simulink model "EPT"  (R2019b)
settings: Solver=FixedStepDiscrete  StartTime=0.0  StopTime=5  FixedStep=0.005  RelTol=1e-3  EnableMultiTasking=on
PreLoadFcn:
  | try, model_open; catch, disp('Error occurred while executing model pre-load callback: model_open.m'); disp('Please assure that the MATLAB working directory is set to the model directory before opening.'); end
InitFcn:
  | try, model_open; catch, end
undefined symbols (not defined in the file or in its folder): Bridge, GCM, H, ln, raptor_get_param_eval, raptor_get_safe_string, raptor_xcp_function
libraries: Raptor_lib x2810, simulink x374, hdlsllib x19
(part 29 of 45)

== system EPT/Foreground_TimeBase_5ms/CAN/CAN3_exec/20CH_TCS/CH1_CH4_Rx/Convert_Byte2Data2 ==
  HighByte : Inport
  LowByte : Inport  Port=2
  Offset : Inport  Port=3
  Factor : Inport  Port=4
  Add2 : Sum
  Add5 : Sum
  Constant10 : Constant  Value=256
  Data Type Conversion10 : DataTypeConversion  OutDataTypeStr=double
  Divide6 : Product  Inputs=**
  Divide9 : Product  Inputs=**
  Data : Outport  VectorParamsAs1DForOutWhenUnconnected=off
  wires:
  Divide6/1 -> Add2/2
  LowByte/1 -> Add2/1
  Add5/1 -> Data Type Conversion10/1
  HighByte/1 -> Divide6/1
  Constant10/1 -> Divide6/2
  Divide9/1 -> Add5/1
  Add2/1 -> Divide9/1
  Data Type Conversion10/1 -> Data/1
  Factor/1 -> Divide9/2
  Offset/1 -> Add5/2

== system EPT/Foreground_TimeBase_5ms/CAN/CAN3_exec/20CH_TCS/CH1_CH4_Rx/Convert_Byte2Data3 ==
  HighByte : Inport
  LowByte : Inport  Port=2
  Offset : Inport  Port=3
  Factor : Inport  Port=4
  Add2 : Sum
  Add5 : Sum
  Constant10 : Constant  Value=256
  Data Type Conversion10 : DataTypeConversion  OutDataTypeStr=double
  Divide6 : Product  Inputs=**
  Divide9 : Product  Inputs=**
  Data : Outport  VectorParamsAs1DForOutWhenUnconnected=off
  wires:
  Offset/1 -> Add5/2
  Factor/1 -> Divide9/2
  Data Type Conversion10/1 -> Data/1
  Add2/1 -> Divide9/1
  Divide9/1 -> Add5/1
  Constant10/1 -> Divide6/2
  HighByte/1 -> Divide6/1
  Add5/1 -> Data Type Conversion10/1
  LowByte/1 -> Add2/1
  Divide6/1 -> Add2/2

== system EPT/Foreground_TimeBase_5ms/CAN/CAN3_exec/20CH_TCS/CH5_CH8_Rx/Convert_Byte2Data ==
  HighByte : Inport
  LowByte : Inport  Port=2
  Offset : Inport  Port=3
  Factor : Inport  Port=4
  Add2 : Sum
  Add5 : Sum
  Constant10 : Constant  Value=256
  Data Type Conversion10 : DataTypeConversion  OutDataTypeStr=double
  Divide6 : Product  Inputs=**
  Divide9 : Product  Inputs=**
  Data : Outport  VectorParamsAs1DForOutWhenUnconnected=off
  wires:
  Divide6/1 -> Add2/2
  LowByte/1 -> Add2/1
  Add5/1 -> Data Type Conversion10/1
  HighByte/1 -> Divide6/1
  Constant10/1 -> Divide6/2
  Divide9/1 -> Add5/1
  Add2/1 -> Divide9/1
  Data Type Conversion10/1 -> Data/1
  Factor/1 -> Divide9/2
  Offset/1 -> Add5/2

== system EPT/Foreground_TimeBase_5ms/CAN/CAN3_exec/20CH_TCS/CH5_CH8_Rx/Convert_Byte2Data1 ==
  HighByte : Inport
  LowByte : Inport  Port=2
  Offset : Inport  Port=3
  Factor : Inport  Port=4
  Add2 : Sum
  Add5 : Sum
  Constant10 : Constant  Value=256
  Data Type Conversion10 : DataTypeConversion  OutDataTypeStr=double
  Divide6 : Product  Inputs=**
  Divide9 : Product  Inputs=**
  Data : Outport  VectorParamsAs1DForOutWhenUnconnected=off
  wires:
  Offset/1 -> Add5/2
  Factor/1 -> Divide9/2
  Data Type Conversion10/1 -> Data/1
  Add2/1 -> Divide9/1
  Divide9/1 -> Add5/1
  Constant10/1 -> Divide6/2
  HighByte/1 -> Divide6/1
  Add5/1 -> Data Type Conversion10/1
  LowByte/1 -> Add2/1
  Divide6/1 -> Add2/2

== system EPT/Foreground_TimeBase_5ms/CAN/CAN3_exec/20CH_TCS/CH5_CH8_Rx/Convert_Byte2Data2 ==
  HighByte : Inport
  LowByte : Inport  Port=2
  Offset : Inport  Port=3
  Factor : Inport  Port=4
  Add2 : Sum
  Add5 : Sum
  Constant10 : Constant  Value=256
  Data Type Conversion10 : DataTypeConversion  OutDataTypeStr=double
  Divide6 : Product  Inputs=**
  Divide9 : Product  Inputs=**
  Data : Outport  VectorParamsAs1DForOutWhenUnconnected=off
  wires:
  Divide6/1 -> Add2/2
  LowByte/1 -> Add2/1
  Add5/1 -> Data Type Conversion10/1
  HighByte/1 -> Divide6/1
  Constant10/1 -> Divide6/2
  Divide9/1 -> Add5/1
  Add2/1 -> Divide9/1
  Data Type Conversion10/1 -> Data/1
  Factor/1 -> Divide9/2
  Offset/1 -> Add5/2

== system EPT/Foreground_TimeBase_5ms/CAN/CAN3_exec/20CH_TCS/CH5_CH8_Rx/Convert_Byte2Data3 ==
  HighByte : Inport
  LowByte : Inport  Port=2
  Offset : Inport  Port=3
  Factor : Inport  Port=4
  Add2 : Sum
  Add5 : Sum
  Constant10 : Constant  Value=256
  Data Type Conversion10 : DataTypeConversion  OutDataTypeStr=double
  Divide6 : Product  Inputs=**
  Divide9 : Product  Inputs=**
  Data : Outport  VectorParamsAs1DForOutWhenUnconnected=off
  wires:
  Offset/1 -> Add5/2
  Factor/1 -> Divide9/2
  Data Type Conversion10/1 -> Data/1
  Add2/1 -> Divide9/1
  Divide9/1 -> Add5/1
  Constant10/1 -> Divide6/2
  HighByte/1 -> Divide6/1
  Add5/1 -> Data Type Conversion10/1
  LowByte/1 -> Add2/1
  Divide6/1 -> Add2/2

== system EPT/Foreground_TimeBase_5ms/CAN/CAN3_exec/20CH_TCS/CH9_CH12_Rx/Convert_Byte2Data ==
  HighByte : Inport
  LowByte : Inport  Port=2
  Offset : Inport  Port=3
  Factor : Inport  Port=4
  Add2 : Sum
  Add5 : Sum
  Constant10 : Constant  Value=256
  Data Type Conversion10 : DataTypeConversion  OutDataTypeStr=double
  Divide6 : Product  Inputs=**
  Divide9 : Product  Inputs=**
  Data : Outport  VectorParamsAs1DForOutWhenUnconnected=off
  wires:
  Divide6/1 -> Add2/2
  LowByte/1 -> Add2/1
  Add5/1 -> Data Type Conversion10/1
  HighByte/1 -> Divide6/1
  Constant10/1 -> Divide6/2
  Divide9/1 -> Add5/1
  Add2/1 -> Divide9/1
  Data Type Conversion10/1 -> Data/1
  Factor/1 -> Divide9/2
  Offset/1 -> Add5/2

== system EPT/Foreground_TimeBase_5ms/CAN/CAN3_exec/20CH_TCS/CH9_CH12_Rx/Convert_Byte2Data1 ==
  HighByte : Inport
  LowByte : Inport  Port=2
  Offset : Inport  Port=3
  Factor : Inport  Port=4
  Add2 : Sum
  Add5 : Sum
  Constant10 : Constant  Value=256
  Data Type Conversion10 : DataTypeConversion  OutDataTypeStr=double
  Divide6 : Product  Inputs=**
  Divide9 : Product  Inputs=**
  Data : Outport  VectorParamsAs1DForOutWhenUnconnected=off
  wires:
  Offset/1 -> Add5/2
  Factor/1 -> Divide9/2
  Data Type Conversion10/1 -> Data/1
  Add2/1 -> Divide9/1
  Divide9/1 -> Add5/1
  Constant10/1 -> Divide6/2
  HighByte/1 -> Divide6/1
  Add5/1 -> Data Type Conversion10/1
  LowByte/1 -> Add2/1
  Divide6/1 -> Add2/2

== system EPT/Foreground_TimeBase_5ms/CAN/CAN3_exec/20CH_TCS/CH9_CH12_Rx/Convert_Byte2Data2 ==
  HighByte : Inport
  LowByte : Inport  Port=2
  Offset : Inport  Port=3
  Factor : Inport  Port=4
  Add2 : Sum
  Add5 : Sum
  Constant10 : Constant  Value=256
  Data Type Conversion10 : DataTypeConversion  OutDataTypeStr=double
  Divide6 : Product  Inputs=**
  Divide9 : Product  Inputs=**
  Data : Outport  VectorParamsAs1DForOutWhenUnconnected=off
  wires:
  Divide6/1 -> Add2/2
  LowByte/1 -> Add2/1
  Add5/1 -> Data Type Conversion10/1
  HighByte/1 -> Divide6/1
  Constant10/1 -> Divide6/2
  Divide9/1 -> Add5/1
  Add2/1 -> Divide9/1
  Data Type Conversion10/1 -> Data/1
  Factor/1 -> Divide9/2
  Offset/1 -> Add5/2

== system EPT/Foreground_TimeBase_5ms/CAN/CAN3_exec/20CH_TCS/CH9_CH12_Rx/Convert_Byte2Data3 ==
  HighByte : Inport
  LowByte : Inport  Port=2
  Offset : Inport  Port=3
  Factor : Inport  Port=4
  Add2 : Sum
  Add5 : Sum
  Constant10 : Constant  Value=256
  Data Type Conversion10 : DataTypeConversion  OutDataTypeStr=double
  Divide6 : Product  Inputs=**
  Divide9 : Product  Inputs=**
  Data : Outport  VectorParamsAs1DForOutWhenUnconnected=off
  wires:
  Offset/1 -> Add5/2
  Factor/1 -> Divide9/2
  Data Type Conversion10/1 -> Data/1
  Add2/1 -> Divide9/1
  Divide9/1 -> Add5/1
  Constant10/1 -> Divide6/2
  HighByte/1 -> Divide6/1
  Add5/1 -> Data Type Conversion10/1
  LowByte/1 -> Add2/1
  Divide6/1 -> Add2/2

== system EPT/Foreground_TimeBase_5ms/CAN/CAN3_exec/20CH_TCS/CountTrigger/CycleTrigger ==
  In1 : Inport
  In2 : Inport  Port=2
  Add : Sum
  Add1 : Sum
  Add2 : Sum  Inputs=+-
  Constant1 : Constant
  Constant2 : Constant  Value=0
  Constant3 : Constant
  Data Type Conversion1 : DataTypeConversion
  Data Type Conversion2 : DataTypeConversion
  Display : Display
  Relational Operator1 : RelationalOperator  OutDataTypeStr=boolean  RndMeth=Simplest
  Scope : Scope
  Scope1 : Scope
  Scope2 : Scope
  Switch : Switch  Threshold=1
  Unit Delay : UnitDelay  SampleTime=-1  HasFrameUpgradeWarning=on
  Unit Delay1 : UnitDelay  SampleTime=-1  HasFrameUpgradeWarning=on
  Trigger : Outport  VectorParamsAs1DForOutWhenUnconnected=off
  wires:
  Constant3/1 -> Add2/2
  In2/1 -> Add2/1
  Add2/1 -> Data Type Conversion1/1
  Data Type Conversion2/1 -> Switch/2, Add/2
  Constant2/1 -> Switch/3
  Data Type Conversion1/1 -> Relational Operator1/2
  Relational Operator1/1 -> Trigger/1, Scope2/1
  Constant1/1 -> Add1/2
  Unit Delay1/1 -> Add1/1
  Add1/1 -> Display/1, Unit Delay1/1, Scope/1
  Switch/1 -> Unit Delay/1, Scope1/1, Relational Operator1/1
  Unit Delay/1 -> Add/1
  In1/1 -> Data Type Conversion2/1
  Add/1 -> Switch/1

== system EPT/Foreground_TimeBase_5ms/CAN/CAN3_exec/DCDC/CountTrigger/CycleTrigger ==
  In1 : Inport
  In2 : Inport  Port=2
  Add : Sum
  Add1 : Sum
  Add2 : Sum  Inputs=+-
  Constant1 : Constant
  Constant2 : Constant  Value=0
  Constant3 : Constant
  Data Type Conversion1 : DataTypeConversion
  Data Type Conversion2 : DataTypeConversion
  Display : Display
  Relational Operator1 : RelationalOperator  OutDataTypeStr=boolean  RndMeth=Simplest
  Scope : Scope
  Scope1 : Scope
  Scope2 : Scope
  Switch : Switch  Threshold=1
  Unit Delay : UnitDelay  SampleTime=-1  HasFrameUpgradeWarning=on
  Unit Delay1 : UnitDelay  SampleTime=-1  HasFrameUpgradeWarning=on
  Trigger : Outport  VectorParamsAs1DForOutWhenUnconnected=off
  wires:
  Constant3/1 -> Add2/2
  In2/1 -> Add2/1
  Add2/1 -> Data Type Conversion1/1
  Data Type Conversion2/1 -> Switch/2, Add/2
  Constant2/1 -> Switch/3
  Data Type Conversion1/1 -> Relational Operator1/2
  Relational Operator1/1 -> Trigger/1, Scope2/1
  Constant1/1 -> Add1/2
  Unit Delay1/1 -> Add1/1
  Add1/1 -> Display/1, Unit Delay1/1, Scope/1
  Switch/1 -> Unit Delay/1, Scope1/1, Relational Operator1/1
  Unit Delay/1 -> Add/1
  In1/1 -> Data Type Conversion2/1
  Add/1 -> Switch/1

== system EPT/Foreground_TimeBase_5ms/CAN/CAN3_exec/DCDC/DCDC_RX_0x180XF45D /Convert_Byte2Data1 ==
  HighByte : Inport
  LowByte : Inport  Port=2
  Offset : Inport  Port=3
  Factor : Inport  Port=4
  Add2 : Sum
  Add5 : Sum
  Constant10 : Constant  Value=256
  Data Type Conversion10 : DataTypeConversion  OutDataTypeStr=double
  Divide6 : Product  Inputs=**
  Divide9 : Product  Inputs=**
  Data : Outport  VectorParamsAs1DForOutWhenUnconnected=off
  wires:
  Offset/1 -> Add5/2
  Factor/1 -> Divide9/2
  Data Type Conversion10/1 -> Data/1
  Add2/1 -> Divide9/1
  Divide9/1 -> Add5/1
  Constant10/1 -> Divide6/2
  HighByte/1 -> Divide6/1
  Add5/1 -> Data Type Conversion10/1
  LowByte/1 -> Add2/1
  Divide6/1 -> Add2/2

== system EPT/Foreground_TimeBase_5ms/CAN/CAN3_exec/DCDC/DCDC_RX_0x180XF45D /Convert_Byte2Data2 ==
  HighByte : Inport
  LowByte : Inport  Port=2
  Offset : Inport  Port=3
  Factor : Inport  Port=4
  Add2 : Sum
  Add5 : Sum
  Constant10 : Constant  Value=256
  Data Type Conversion10 : DataTypeConversion  OutDataTypeStr=double
  Divide6 : Product  Inputs=**
  Divide9 : Product  Inputs=**
  Data : Outport  VectorParamsAs1DForOutWhenUnconnected=off
  wires:
  Divide6/1 -> Add2/2
  LowByte/1 -> Add2/1
  Add5/1 -> Data Type Conversion10/1
  HighByte/1 -> Divide6/1
  Constant10/1 -> Divide6/2
  Divide9/1 -> Add5/1
  Add2/1 -> Divide9/1
  Data Type Conversion10/1 -> Data/1
  Factor/1 -> Divide9/2
  Offset/1 -> Add5/2

== system EPT/Foreground_TimeBase_5ms/CAN/CAN3_exec/DCDC/DCDC_RX_0x180XF45D /Convert_Byte2Data3 ==
  HighByte : Inport
  LowByte : Inport  Port=2
  Offset : Inport  Port=3
  Factor : Inport  Port=4
  Add2 : Sum
  Add5 : Sum
  Constant10 : Constant  Value=256
  Data Type Conversion10 : DataTypeConversion  OutDataTypeStr=double
  Divide6 : Product  Inputs=**
  Divide9 : Product  Inputs=**
  Data : Outport  VectorParamsAs1DForOutWhenUnconnected=off
  wires:
  Divide6/1 -> Add2/2
  LowByte/1 -> Add2/1
  Add5/1 -> Data Type Conversion10/1
  HighByte/1 -> Divide6/1
  Constant10/1 -> Divide6/2
  Divide9/1 -> Add5/1
  Add2/1 -> Divide9/1
  Data Type Conversion10/1 -> Data/1
  Factor/1 -> Divide9/2
  Offset/1 -> Add5/2

== system EPT/Foreground_TimeBase_5ms/CAN/CAN3_exec/HyPer9_MCU/CountTrigger2/CycleTrigger ==
  In1 : Inport
  In2 : Inport  Port=2
  Add : Sum
  Add1 : Sum
  Add2 : Sum  Inputs=+-
  Constant1 : Constant
  Constant2 : Constant  Value=0
  Constant3 : Constant
  Data Type Conversion1 : DataTypeConversion
  Data Type Conversion2 : DataTypeConversion
  Display : Display
  Relational Operator1 : RelationalOperator  OutDataTypeStr=boolean  RndMeth=Simplest
  Scope : Scope
  Scope1 : Scope
  Scope2 : Scope
  Switch : Switch  Threshold=1
  Unit Delay : UnitDelay  SampleTime=-1  HasFrameUpgradeWarning=on
  Unit Delay1 : UnitDelay  SampleTime=-1  HasFrameUpgradeWarning=on
  Trigger : Outport  VectorParamsAs1DForOutWhenUnconnected=off
  wires:
  Add/1 -> Switch/1
  In1/1 -> Data Type Conversion2/1
  Unit Delay/1 -> Add/1
  Switch/1 -> Relational Operator1/1, Scope1/1, Unit Delay/1
  Add1/1 -> Scope/1, Unit Delay1/1, Display/1
  Unit Delay1/1 -> Add1/1
  Constant1/1 -> Add1/2
  Relational Operator1/1 -> Scope2/1, Trigger/1
  Data Type Conversion1/1 -> Relational Operator1/2
  Constant2/1 -> Switch/3
  Data Type Conversion2/1 -> Add/2, Switch/2
  Add2/1 -> Data Type Conversion1/1
  In2/1 -> Add2/1
  Constant3/1 -> Add2/2

== system EPT/Foreground_TimeBase_5ms/CAN/CAN3_exec/HyPer9_MCU/RPDO1/Byte1 ==
  Bit Shift1 : hdlsllib/Logic and Bit Operations/Bit Shift  mode=Shift Left Logical  N=1
  Bit Shift2 : hdlsllib/Logic and Bit Operations/Bit Shift  mode=Shift Left Logical  N=2
  Bit Shift3 : hdlsllib/Logic and Bit Operations/Bit Shift  mode=Shift Left Logical  N=3
  Bit Shift4 : hdlsllib/Logic and Bit Operations/Bit Shift  mode=Shift Left Logical  N=4
  Bit Shift5 : hdlsllib/Logic and Bit Operations/Bit Shift  mode=Shift Left Logical  N=5
  Bit Shift6 : hdlsllib/Logic and Bit Operations/Bit Shift  mode=Shift Left Logical  N=6
  Bit Shift7 : hdlsllib/Logic and Bit Operations/Bit Shift  mode=Shift Left Logical  N=7
  Bitwise OR : simulink/Logic and Bit Operations/Bitwise Operator  logicop=OR  UseBitMask=off  NumInputPorts=8  BitMask=bin2dec('11011001')  BitMaskRealWorld=Stored Integer
  Data Type Conversion{1..9} (9 alike) : DataTypeConversion  OutDataTypeStr=uint8
  "First Sw Reset Request " : Constant  Value=0  OutDataTypeStr=uint8
  IsPositive{1..7} (7 alike) : simulink/Logic and Bit Operations/Compare To Zero  relop=>  OutDataTypeStr=boolean
  Request for Digital Output 1 : Constant  Value=0  OutDataTypeStr=uint8
  Request for Digital Output 2 : Constant  Value=0  OutDataTypeStr=uint8
  Request for Driver Output 1 in Voltage Mode : Constant  Value=0  OutDataTypeStr=uint8
  Request for Driver Output 2 in Voltage Mode : Constant  Value=0  OutDataTypeStr=uint8
  Request for Driver Output 3 in Voltage Mode : Constant  Value=0  OutDataTypeStr=uint8
  Request for Driver Output 4 in Voltage Mode (only Control Mode allowed) : Constant  Value=0  OutDataTypeStr=uint8
  Second Sw Reset Request : Constant  Value=0  OutDataTypeStr=uint8
  Byte : Outport
  wires:
  IsPositive6/1 -> Data Type Conversion7/1
  Request for Driver Output 4 in Voltage Mode (only Control Mode allowed)/1 -> IsPositive7/1
  Data Type Conversion2/1 -> Bitwise OR/1
  IsPositive7/1 -> Data Type Conversion8/1
  IsPositive3/1 -> Data Type Conversion4/1
  Request for Driver Output 1 in Voltage Mode/1 -> IsPositive2/1
  Bit Shift4/1 -> Bitwise OR/5
  Bit Shift6/1 -> Bitwise OR/7
  IsPositive2/1 -> Data Type Conversion3/1
  "First Sw Reset Request "/1 -> IsPositive5/1
  IsPositive5/1 -> Data Type Conversion6/1
  Bit Shift3/1 -> Bitwise OR/4
  Data Type Conversion5/1 -> Bit Shift4/1
  Data Type Conversion8/1 -> Bit Shift7/1
  Bit Shift7/1 -> Bitwise OR/8
  Request for Digital Output 1/1 -> Data Type Conversion2/1
  Bit Shift2/1 -> Bitwise OR/3
  Bitwise OR/1 -> Data Type Conversion9/1
  Data Type Conversion4/1 -> Bit Shift3/1
  Request for Digital Output 2/1 -> IsPositive1/1
  Data Type Conversion7/1 -> Bit Shift6/1
  IsPositive1/1 -> Data Type Conversion1/1
  Data Type Conversion1/1 -> Bit Shift1/1
  Bit Shift5/1 -> Bitwise OR/6
  Request for Driver Output 2 in Voltage Mode/1 -> IsPositive3/1
  Second Sw Reset Request/1 -> IsPositive6/1
  IsPositive4/1 -> Data Type Conversion5/1
  Request for Driver Output 3 in Voltage Mode/1 -> IsPositive4/1
  Data Type Conversion9/1 -> Byte/1
  Data Type Conversion6/1 -> Bit Shift5/1
  Bit Shift1/1 -> Bitwise OR/2
  Data Type Conversion3/1 -> Bit Shift2/1

== system EPT/Foreground_TimeBase_5ms/CAN/CAN3_exec/HyPer9_MCU/RPDO1/Convert_Data2Byte ==
  Data : Inport
  Factor : Inport  Port=2
  Offset : Inport  Port=3
  Add : Sum
  Bitwise Operator : simulink/Logic and Bit Operations/Bitwise Operator  logicop=AND  UseBitMask=on  BitMask=bin2dec('1111111100000000')  BitMaskRealWorld=Stored Integer
  Bitwise Operator1 : simulink/Logic and Bit Operations/Bitwise Operator  logicop=AND  UseBitMask=on  BitMask=bin2dec('0000000011111111')  BitMaskRealWorld=Stored Integer
  Compare To Zero : simulink/Logic and Bit Operations/Compare To Zero  relop=~=  OutDataTypeStr=boolean
  Constant : Constant
  Data Type Conversion : DataTypeConversion
  Data Type Conversion1 : DataTypeConversion  OutDataTypeStr=uint16
  Data Type Conversion2 : DataTypeConversion
  Display : Display
      settings: Format=hex (Stored Integer)
  Divide : Product  Inputs=**
  Shift Arithmetic : ArithShift  BitShiftNumber=8  BitShiftDirection=Right
  Switch : Switch  Criteria=u2 > Threshold
  LowByte : Outport  VectorParamsAs1DForOutWhenUnconnected=off
  HighByte : Outport  Port=2  VectorParamsAs1DForOutWhenUnconnected=off
  wires:
  Compare To Zero/1 -> Switch/2
  Factor/1 -> Switch/1, Compare To Zero/1
  Data Type Conversion2/1 -> HighByte/1
  Data Type Conversion/1 -> LowByte/1
  Constant/1 -> Switch/3
  Switch/1 -> Divide/2
  Bitwise Operator/1 -> Shift Arithmetic/1
  Offset/1 -> Add/2
  Shift Arithmetic/1 -> Data Type Conversion2/1
  Bitwise Operator1/1 -> Data Type Conversion/1
  Data Type Conversion1/1 -> Bitwise Operator/1, Display/1, Bitwise Operator1/1
  Divide/1 -> Add/1
  Data/1 -> Divide/1
  Add/1 -> Data Type Conversion1/1

== system EPT/Foreground_TimeBase_5ms/CAN/CAN3_exec/HyPer9_MCU/RPDO1/Convert_Data2Byte1 ==
  Data : Inport
  Factor : Inport  Port=2
  Offset : Inport  Port=3
  Add : Sum
  Bitwise Operator : simulink/Logic and Bit Operations/Bitwise Operator  logicop=AND  UseBitMask=on  BitMask=bin2dec('1111111100000000')  BitMaskRealWorld=Stored Integer
  Bitwise Operator1 : simulink/Logic and Bit Operations/Bitwise Operator  logicop=AND  UseBitMask=on  BitMask=bin2dec('0000000011111111')  BitMaskRealWorld=Stored Integer
  Compare To Zero : simulink/Logic and Bit Operations/Compare To Zero  relop=~=  OutDataTypeStr=boolean
  Constant : Constant
  Data Type Conversion : DataTypeConversion
  Data Type Conversion1 : DataTypeConversion  OutDataTypeStr=uint16
  Data Type Conversion2 : DataTypeConversion
  Display : Display
      settings: Format=hex (Stored Integer)
  Divide : Product  Inputs=**
  Shift Arithmetic : ArithShift  BitShiftNumber=8  BitShiftDirection=Right
  Switch : Switch  Criteria=u2 > Threshold
  LowByte : Outport  VectorParamsAs1DForOutWhenUnconnected=off
  HighByte : Outport  Port=2  VectorParamsAs1DForOutWhenUnconnected=off
  wires:
  Add/1 -> Data Type Conversion1/1
  Data/1 -> Divide/1
  Divide/1 -> Add/1
  Data Type Conversion1/1 -> Bitwise Operator1/1, Display/1, Bitwise Operator/1
  Bitwise Operator1/1 -> Data Type Conversion/1
  Shift Arithmetic/1 -> Data Type Conversion2/1
  Offset/1 -> Add/2
  Bitwise Operator/1 -> Shift Arithmetic/1
  Switch/1 -> Divide/2
  Constant/1 -> Switch/3
  Data Type Conversion/1 -> LowByte/1
  Data Type Conversion2/1 -> HighByte/1
  Factor/1 -> Compare To Zero/1, Switch/1
  Compare To Zero/1 -> Switch/2

== system EPT/Foreground_TimeBase_5ms/CAN/CAN3_exec/HyPer9_MCU/RPDO1/Convert_Data2Byte2 ==
  Data : Inport
  Factor : Inport  Port=2
  Offset : Inport  Port=3
  Add : Sum
  Bitwise Operator : simulink/Logic and Bit Operations/Bitwise Operator  logicop=AND  UseBitMask=on  BitMask=bin2dec('1111111100000000')  BitMaskRealWorld=Stored Integer
  Bitwise Operator1 : simulink/Logic and Bit Operations/Bitwise Operator  logicop=AND  UseBitMask=on  BitMask=bin2dec('0000000011111111')  BitMaskRealWorld=Stored Integer
  Compare To Zero : simulink/Logic and Bit Operations/Compare To Zero  relop=~=  OutDataTypeStr=boolean
  Constant : Constant
  Data Type Conversion : DataTypeConversion
  Data Type Conversion1 : DataTypeConversion  OutDataTypeStr=uint16
  Data Type Conversion2 : DataTypeConversion
  Display : Display
      settings: Format=hex (Stored Integer)
  Divide : Product  Inputs=**
  Shift Arithmetic : ArithShift  BitShiftNumber=8  BitShiftDirection=Right
  Switch : Switch  Criteria=u2 > Threshold
  LowByte : Outport  VectorParamsAs1DForOutWhenUnconnected=off
  HighByte : Outport  Port=2  VectorParamsAs1DForOutWhenUnconnected=off
  wires:
  Compare To Zero/1 -> Switch/2
  Factor/1 -> Switch/1, Compare To Zero/1
  Data Type Conversion2/1 -> HighByte/1
  Data Type Conversion/1 -> LowByte/1
  Constant/1 -> Switch/3
  Switch/1 -> Divide/2
  Bitwise Operator/1 -> Shift Arithmetic/1
  Offset/1 -> Add/2
  Shift Arithmetic/1 -> Data Type Conversion2/1
  Bitwise Operator1/1 -> Data Type Conversion/1
  Data Type Conversion1/1 -> Bitwise Operator/1, Display/1, Bitwise Operator1/1
  Divide/1 -> Add/1
  Data/1 -> Divide/1
  Add/1 -> Data Type Conversion1/1

== system EPT/Foreground_TimeBase_5ms/CAN/CAN3_exec/HyPer9_MCU/RPDO2/Byte5 ==
  Bit Shift1 : hdlsllib/Logic and Bit Operations/Bit Shift  mode=Shift Left Logical  N=2
  Bit Shift2 : hdlsllib/Logic and Bit Operations/Bit Shift  mode=Shift Left Logical  N=3
  Bit Shift3 : hdlsllib/Logic and Bit Operations/Bit Shift  mode=Shift Left Logical  N=4
  Bit Shift4 : hdlsllib/Logic and Bit Operations/Bit Shift  mode=Shift Left Logical  N=5
  Bit Shift5 : hdlsllib/Logic and Bit Operations/Bit Shift  mode=Shift Left Logical  N=6
  Bitwise Operator1 : simulink/Logic and Bit Operations/Bitwise Operator  logicop=AND  UseBitMask=on  BitMask=bin2dec('11')  BitMaskRealWorld=Stored Integer
  Bitwise OR : simulink/Logic and Bit Operations/Bitwise Operator  logicop=OR  UseBitMask=off  NumInputPorts=6  BitMask=bin2dec('11011001')  BitMaskRealWorld=Stored Integer
  Data Type Conversion{1..6,9} (7 alike) : DataTypeConversion  OutDataTypeStr=uint8
  Display : Display
      settings: Format=binary (Stored Integer)
  IsPositive{1..5} (5 alike) : simulink/Logic and Bit Operations/Compare To Zero  relop=>  OutDataTypeStr=boolean
  "Motor 1 - Control Mode Request " : Constant  Value=2  OutDataTypeStr=uint8
  raptor_adjustment : Raptor_lib/Data Storage/raptor_adjustment  paramName='Cal_Motor1_Motor1_PWM_Output_Enable_Request'  nameSource=Parameter  initValue=0.00  dataType=double  storage=Calibration  calDispType=Number  calEnum={'False', 'True'}  calGain=1.0  calOffset=0.0  calMax=9  calMin=-inf  calFormat='-1'  calUnit=''  calHelp=''  calAccess=1  calFunction=raptor_xcp_function(gcb)  calDispHeaders=off  calColHeaders={'Col1' 'Col2' 'Col3'}  calRowHeaders={'Row1' 'Row2' 'Row3'}
      settings: SourceProductName=Raptor
  raptor_adjustment1 : Raptor_lib/Data Storage/raptor_adjustment  paramName='Cal_Motor1_Reference_Torque_Enable_Request'  nameSource=Parameter  initValue=0.00  dataType=double  storage=Calibration  calDispType=Number  calEnum={'False', 'True'}  calGain=1.0  calOffset=0.0  calMax=9  calMin=-inf  calFormat='-1'  calUnit=''  calHelp=''  calAccess=1  calFunction=raptor_xcp_function(gcb)  calDispHeaders=off  calColHeaders={'Col1' 'Col2' 'Col3'}  calRowHeaders={'Row1' 'Row2' 'Row3'}
      settings: SourceProductName=Raptor
  raptor_adjustment2 : Raptor_lib/Data Storage/raptor_adjustment  paramName='Cal_Motor1_Emergency_Stop_Request'  nameSource=Parameter  initValue=0.00  dataType=double  storage=Calibration  calDispType=Number  calEnum={'False', 'True'}  calGain=1.0  calOffset=0.0  calMax=9  calMin=-inf  calFormat='-1'  calUnit=''  calHelp=''  calAccess=1  calFunction=raptor_xcp_function(gcb)  calDispHeaders=off  calColHeaders={'Col1' 'Col2' 'Col3'}  calRowHeaders={'Row1' 'Row2' 'Row3'}
      settings: SourceProductName=Raptor
  raptor_adjustment3 : Raptor_lib/Data Storage/raptor_adjustment  paramName='Cal_Motor1_Safe_Stop_Request'  nameSource=Parameter  initValue=0.00  dataType=double  storage=Calibration  calDispType=Number  calEnum={'False', 'True'}  calGain=1.0  calOffset=0.0  calMax=9  calMin=-inf  calFormat='-1'  calUnit=''  calHelp=''  calAccess=1  calFunction=raptor_xcp_function(gcb)  calDispHeaders=off  calColHeaders={'Col1' 'Col2' 'Col3'}  calRowHeaders={'Row1' 'Row2' 'Row3'}
      settings: SourceProductName=Raptor
  raptor_adjustment4 : Raptor_lib/Data Storage/raptor_adjustment  paramName='Cal_Motor1_Speed_Limit_Request'  nameSource=Parameter  initValue=0.00  dataType=double  storage=Calibration  calDispType=Number  calEnum={'False', 'True'}  calGain=1.0  calOffset=0.0  calMax=9  calMin=-inf  calFormat='-1'  calUnit=''  calHelp=''  calAccess=1  calFunction=raptor_xcp_function(gcb)  calDispHeaders=off  calColHeaders={'Col1' 'Col2' 'Col3'}  calRowHeaders={'Row1' 'Row2' 'Row3'}
      settings: SourceProductName=Raptor
  Byte : Outport
  wires:
  Data Type Conversion2/1 -> Bitwise OR/1
  IsPositive3/1 -> Data Type Conversion4/1
  raptor_adjustment1/1 -> IsPositive2/1
  Bit Shift4/1 -> Bitwise OR/5
  IsPositive2/1 -> Data Type Conversion3/1
  raptor_adjustment4/1 -> IsPositive5/1
  IsPositive5/1 -> Data Type Conversion6/1
  Bit Shift3/1 -> Bitwise OR/4
  Data Type Conversion5/1 -> Bit Shift4/1
  "Motor 1 - Control Mode Request "/1 -> Bitwise Operator1/1
  Bit Shift2/1 -> Bitwise OR/3
  Bitwise OR/1 -> Data Type Conversion9/1
  Data Type Conversion4/1 -> Bit Shift3/1
  raptor_adjustment/1 -> IsPositive1/1
  IsPositive1/1 -> Data Type Conversion1/1
  Data Type Conversion1/1 -> Bit Shift1/1
  Bit Shift5/1 -> Bitwise OR/6
  raptor_adjustment2/1 -> IsPositive3/1
  IsPositive4/1 -> Data Type Conversion5/1
  raptor_adjustment3/1 -> IsPositive4/1
  Data Type Conversion9/1 -> Display/1, Byte/1
  Data Type Conversion6/1 -> Bit Shift5/1
  Bit Shift1/1 -> Bitwise OR/2
  Data Type Conversion3/1 -> Bit Shift2/1
  Bitwise Operator1/1 -> Data Type Conversion2/1

== system EPT/Foreground_TimeBase_5ms/CAN/CAN3_exec/HyPer9_MCU/RPDO2/Convert_Data2Byte ==
  Data : Inport
  Factor : Inport  Port=2
  Offset : Inport  Port=3
  Add : Sum
  Bitwise Operator : simulink/Logic and Bit Operations/Bitwise Operator  logicop=AND  UseBitMask=on  BitMask=bin2dec('1111111100000000')  BitMaskRealWorld=Stored Integer
  Bitwise Operator1 : simulink/Logic and Bit Operations/Bitwise Operator  logicop=AND  UseBitMask=on  BitMask=bin2dec('0000000011111111')  BitMaskRealWorld=Stored Integer
  Compare To Zero : simulink/Logic and Bit Operations/Compare To Zero  relop=~=  OutDataTypeStr=boolean
  Constant : Constant
  Data Type Conversion : DataTypeConversion
  Data Type Conversion1 : DataTypeConversion  OutDataTypeStr=uint16
  Data Type Conversion2 : DataTypeConversion
  Display : Display
      settings: Format=hex (Stored Integer)
  Divide : Product  Inputs=**
  Shift Arithmetic : ArithShift  BitShiftNumber=8  BitShiftDirection=Right
  Switch : Switch  Criteria=u2 > Threshold
  LowByte : Outport  VectorParamsAs1DForOutWhenUnconnected=off
  HighByte : Outport  Port=2  VectorParamsAs1DForOutWhenUnconnected=off
  wires:
  Add/1 -> Data Type Conversion1/1
  Data/1 -> Divide/1
  Divide/1 -> Add/1
  Data Type Conversion1/1 -> Bitwise Operator1/1, Display/1, Bitwise Operator/1
  Bitwise Operator1/1 -> Data Type Conversion/1
  Shift Arithmetic/1 -> Data Type Conversion2/1
  Offset/1 -> Add/2
  Bitwise Operator/1 -> Shift Arithmetic/1
  Switch/1 -> Divide/2
  Constant/1 -> Switch/3
  Data Type Conversion/1 -> LowByte/1
  Data Type Conversion2/1 -> HighByte/1
  Factor/1 -> Compare To Zero/1, Switch/1
  Compare To Zero/1 -> Switch/2

== system EPT/Foreground_TimeBase_5ms/CAN/CAN3_exec/HyPer9_MCU/RPDO2/Convert_Data2Byte1 ==
  Data : Inport
  Factor : Inport  Port=2
  Offset : Inport  Port=3
  Add : Sum
  Bitwise Operator : simulink/Logic and Bit Operations/Bitwise Operator  logicop=AND  UseBitMask=on  BitMask=bin2dec('1111111100000000')  BitMaskRealWorld=Stored Integer
  Bitwise Operator1 : simulink/Logic and Bit Operations/Bitwise Operator  logicop=AND  UseBitMask=on  BitMask=bin2dec('0000000011111111')  BitMaskRealWorld=Stored Integer
  Compare To Zero : simulink/Logic and Bit Operations/Compare To Zero  relop=~=  OutDataTypeStr=boolean
  Constant : Constant
  Data Type Conversion : DataTypeConversion
  Data Type Conversion1 : DataTypeConversion  OutDataTypeStr=uint16
  Data Type Conversion2 : DataTypeConversion
  Display : Display
      settings: Format=hex (Stored Integer)
  Divide : Product  Inputs=**
  Shift Arithmetic : ArithShift  BitShiftNumber=8  BitShiftDirection=Right
  Switch : Switch  Criteria=u2 > Threshold
  LowByte : Outport  VectorParamsAs1DForOutWhenUnconnected=off
  HighByte : Outport  Port=2  VectorParamsAs1DForOutWhenUnconnected=off
  wires:
  Compare To Zero/1 -> Switch/2
  Factor/1 -> Switch/1, Compare To Zero/1
  Data Type Conversion2/1 -> HighByte/1
  Data Type Conversion/1 -> LowByte/1
  Constant/1 -> Switch/3
  Switch/1 -> Divide/2
  Bitwise Operator/1 -> Shift Arithmetic/1
  Offset/1 -> Add/2
  Shift Arithmetic/1 -> Data Type Conversion2/1
  Bitwise Operator1/1 -> Data Type Conversion/1
  Data Type Conversion1/1 -> Bitwise Operator/1, Display/1, Bitwise Operator1/1
  Divide/1 -> Add/1
  Data/1 -> Divide/1
  Add/1 -> Data Type Conversion1/1

== system EPT/Foreground_TimeBase_5ms/CAN/CAN3_exec/HyPer9_MCU/RPDO2/Convert_Data2Byte2 ==
  Data : Inport
  Factor : Inport  Port=2
  Offset : Inport  Port=3
  Add : Sum
  Bitwise Operator1 : simulink/Logic and Bit Operations/Bitwise Operator  logicop=AND  UseBitMask=on  BitMask=bin2dec('0000000011111111')  BitMaskRealWorld=Stored Integer
  Compare To Zero : simulink/Logic and Bit Operations/Compare To Zero  relop=~=  OutDataTypeStr=boolean
  Constant : Constant
  Data Type Conversion : DataTypeConversion
  Data Type Conversion1 : DataTypeConversion  OutDataTypeStr=uint16
  Display : Display
      settings: Format=hex (Stored Integer)
  Divide : Product  Inputs=**
  Switch : Switch  Criteria=u2 > Threshold
  LowByte : Outport  VectorParamsAs1DForOutWhenUnconnected=off
  wires:
  Add/1 -> Data Type Conversion1/1
  Data/1 -> Divide/1
  Divide/1 -> Add/1
  Data Type Conversion1/1 -> Display/1, Bitwise Operator1/1
  Bitwise Operator1/1 -> Data Type Conversion/1
  Offset/1 -> Add/2
  Switch/1 -> Divide/2
  Constant/1 -> Switch/3
  Data Type Conversion/1 -> LowByte/1
  Factor/1 -> Compare To Zero/1, Switch/1
  Compare To Zero/1 -> Switch/2

== system EPT/Foreground_TimeBase_5ms/CAN/CAN3_exec/HyPer9_MCU/RPDO3/Byte5 ==
  Bit Shift1 : hdlsllib/Logic and Bit Operations/Bit Shift  mode=Shift Left Logical  N=2
  Bit Shift2 : hdlsllib/Logic and Bit Operations/Bit Shift  mode=Shift Left Logical  N=3
  Bit Shift3 : hdlsllib/Logic and Bit Operations/Bit Shift  mode=Shift Left Logical  N=4
  Bit Shift4 : hdlsllib/Logic and Bit Operations/Bit Shift  mode=Shift Left Logical  N=5
  Bit Shift5 : hdlsllib/Logic and Bit Operations/Bit Shift  mode=Shift Left Logical  N=6
  Bitwise Operator1 : simulink/Logic and Bit Operations/Bitwise Operator  logicop=AND  UseBitMask=on  BitMask=bin2dec('11')  BitMaskRealWorld=Stored Integer
  Bitwise OR : simulink/Logic and Bit Operations/Bitwise Operator  logicop=OR  UseBitMask=off  NumInputPorts=6  BitMask=bin2dec('11011001')  BitMaskRealWorld=Stored Integer
  Data Type Conversion{1..6,9} (7 alike) : DataTypeConversion  OutDataTypeStr=uint8
  Display : Display
      settings: Format=binary (Stored Integer)
  IsPositive{1..5} (5 alike) : simulink/Logic and Bit Operations/Compare To Zero  relop=>  OutDataTypeStr=boolean
  "Motor 2 - Control Mode Request " : Constant  Value=0  OutDataTypeStr=uint8
  "Motor 2 - Emergency Stop Request " : Constant  Value=0  OutDataTypeStr=uint8
  "Motor 2 - PWM Output Enable Request " : Constant  Value=0  OutDataTypeStr=uint8
  "Motor 2 - Reference Speed/Torque Enable Request " : Constant  Value=0  OutDataTypeStr=uint8
  "Motor 2 - Safe Stop Request " : Constant  Value=0  OutDataTypeStr=uint8
  "Motor 2 - Speed Limit Request " : Constant  Value=0  OutDataTypeStr=uint8
  Byte : Outport
  wires:
  Bitwise Operator1/1 -> Data Type Conversion2/1
  Data Type Conversion3/1 -> Bit Shift2/1
  Bit Shift1/1 -> Bitwise OR/2
  Data Type Conversion6/1 -> Bit Shift5/1
  Data Type Conversion9/1 -> Byte/1, Display/1
  "Motor 2 - Safe Stop Request "/1 -> IsPositive4/1
  IsPositive4/1 -> Data Type Conversion5/1
  "Motor 2 - Emergency Stop Request "/1 -> IsPositive3/1
  Bit Shift5/1 -> Bitwise OR/6
  Data Type Conversion1/1 -> Bit Shift1/1
  IsPositive1/1 -> Data Type Conversion1/1
  "Motor 2 - PWM Output Enable Request "/1 -> IsPositive1/1
  Data Type Conversion4/1 -> Bit Shift3/1
  Bitwise OR/1 -> Data Type Conversion9/1
  Bit Shift2/1 -> Bitwise OR/3
  "Motor 2 - Control Mode Request "/1 -> Bitwise Operator1/1
  Data Type Conversion5/1 -> Bit Shift4/1
  Bit Shift3/1 -> Bitwise OR/4
  IsPositive5/1 -> Data Type Conversion6/1
  "Motor 2 - Speed Limit Request "/1 -> IsPositive5/1
  IsPositive2/1 -> Data Type Conversion3/1
  Bit Shift4/1 -> Bitwise OR/5
  "Motor 2 - Reference Speed/Torque Enable Request "/1 -> IsPositive2/1
  IsPositive3/1 -> Data Type Conversion4/1
  Data Type Conversion2/1 -> Bitwise OR/1

== system EPT/Foreground_TimeBase_5ms/CAN/CAN3_exec/HyPer9_MCU/RPDO3/Convert_Data2Byte ==
  Data : Inport
  Factor : Inport  Port=2
  Offset : Inport  Port=3
  Add : Sum
  Bitwise Operator : simulink/Logic and Bit Operations/Bitwise Operator  logicop=AND  UseBitMask=on  BitMask=bin2dec('1111111100000000')  BitMaskRealWorld=Stored Integer
  Bitwise Operator1 : simulink/Logic and Bit Operations/Bitwise Operator  logicop=AND  UseBitMask=on  BitMask=bin2dec('0000000011111111')  BitMaskRealWorld=Stored Integer
  Compare To Zero : simulink/Logic and Bit Operations/Compare To Zero  relop=~=  OutDataTypeStr=boolean
  Constant : Constant
  Data Type Conversion : DataTypeConversion
  Data Type Conversion1 : DataTypeConversion  OutDataTypeStr=uint16
  Data Type Conversion2 : DataTypeConversion
  Display : Display
      settings: Format=hex (Stored Integer)
  Divide : Product  Inputs=**
  Shift Arithmetic : ArithShift  BitShiftNumber=8  BitShiftDirection=Right
  Switch : Switch  Criteria=u2 > Threshold
  LowByte : Outport  VectorParamsAs1DForOutWhenUnconnected=off
  HighByte : Outport  Port=2  VectorParamsAs1DForOutWhenUnconnected=off
  wires:
  Compare To Zero/1 -> Switch/2
  Factor/1 -> Switch/1, Compare To Zero/1
  Data Type Conversion2/1 -> HighByte/1
  Data Type Conversion/1 -> LowByte/1
  Constant/1 -> Switch/3
  Switch/1 -> Divide/2
  Bitwise Operator/1 -> Shift Arithmetic/1
  Offset/1 -> Add/2
  Shift Arithmetic/1 -> Data Type Conversion2/1
  Bitwise Operator1/1 -> Data Type Conversion/1
  Data Type Conversion1/1 -> Bitwise Operator/1, Display/1, Bitwise Operator1/1
  Divide/1 -> Add/1
  Data/1 -> Divide/1
  Add/1 -> Data Type Conversion1/1

== system EPT/Foreground_TimeBase_5ms/CAN/CAN3_exec/HyPer9_MCU/RPDO3/Convert_Data2Byte1 ==
  Data : Inport
  Factor : Inport  Port=2
  Offset : Inport  Port=3
  Add : Sum
  Bitwise Operator : simulink/Logic and Bit Operations/Bitwise Operator  logicop=AND  UseBitMask=on  BitMask=bin2dec('1111111100000000')  BitMaskRealWorld=Stored Integer
  Bitwise Operator1 : simulink/Logic and Bit Operations/Bitwise Operator  logicop=AND  UseBitMask=on  BitMask=bin2dec('0000000011111111')  BitMaskRealWorld=Stored Integer
  Compare To Zero : simulink/Logic and Bit Operations/Compare To Zero  relop=~=  OutDataTypeStr=boolean
  Constant : Constant
  Data Type Conversion : DataTypeConversion
  Data Type Conversion1 : DataTypeConversion  OutDataTypeStr=uint16
  Data Type Conversion2 : DataTypeConversion
  Display : Display
      settings: Format=hex (Stored Integer)
  Divide : Product  Inputs=**
  Shift Arithmetic : ArithShift  BitShiftNumber=8  BitShiftDirection=Right
  Switch : Switch  Criteria=u2 > Threshold
  LowByte : Outport  VectorParamsAs1DForOutWhenUnconnected=off
  HighByte : Outport  Port=2  VectorParamsAs1DForOutWhenUnconnected=off
  wires:
  Add/1 -> Data Type Conversion1/1
  Data/1 -> Divide/1
  Divide/1 -> Add/1
  Data Type Conversion1/1 -> Bitwise Operator1/1, Display/1, Bitwise Operator/1
  Bitwise Operator1/1 -> Data Type Conversion/1
  Shift Arithmetic/1 -> Data Type Conversion2/1
  Offset/1 -> Add/2
  Bitwise Operator/1 -> Shift Arithmetic/1
  Switch/1 -> Divide/2
  Constant/1 -> Switch/3
  Data Type Conversion/1 -> LowByte/1
  Data Type Conversion2/1 -> HighByte/1
  Factor/1 -> Compare To Zero/1, Switch/1
  Compare To Zero/1 -> Switch/2

== system EPT/Foreground_TimeBase_5ms/CAN/CAN3_exec/HyPer9_MCU/RPDO3/Convert_Data2Byte2 ==
  Data : Inport
  Factor : Inport  Port=2
  Offset : Inport  Port=3
  Add : Sum
  Bitwise Operator1 : simulink/Logic and Bit Operations/Bitwise Operator  logicop=AND  UseBitMask=on  BitMask=bin2dec('0000000011111111')  BitMaskRealWorld=Stored Integer
  Compare To Zero : simulink/Logic and Bit Operations/Compare To Zero  relop=~=  OutDataTypeStr=boolean
  Constant : Constant
  Data Type Conversion : DataTypeConversion
  Data Type Conversion1 : DataTypeConversion  OutDataTypeStr=uint16
  Display : Display
      settings: Format=hex (Stored Integer)
  Divide : Product  Inputs=**
  Switch : Switch  Criteria=u2 > Threshold
  LowByte : Outport  VectorParamsAs1DForOutWhenUnconnected=off
  wires:
  Add/1 -> Data Type Conversion1/1
  Data/1 -> Divide/1
  Divide/1 -> Add/1
  Data Type Conversion1/1 -> Display/1, Bitwise Operator1/1
  Bitwise Operator1/1 -> Data Type Conversion/1
  Offset/1 -> Add/2
  Switch/1 -> Divide/2
  Constant/1 -> Switch/3
  Data Type Conversion/1 -> LowByte/1
  Factor/1 -> Compare To Zero/1, Switch/1
  Compare To Zero/1 -> Switch/2

== system EPT/Foreground_TimeBase_5ms/CAN/CAN3_exec/HyPer9_MCU/RPDO4/Convert_Data2Byte ==
  Data : Inport
  Factor : Inport  Port=2
  Offset : Inport  Port=3
  Add : Sum
  Bitwise Operator : simulink/Logic and Bit Operations/Bitwise Operator  logicop=AND  UseBitMask=on  BitMask=bin2dec('1111111100000000')  BitMaskRealWorld=Stored Integer
  Bitwise Operator1 : simulink/Logic and Bit Operations/Bitwise Operator  logicop=AND  UseBitMask=on  BitMask=bin2dec('0000000011111111')  BitMaskRealWorld=Stored Integer
  Compare To Zero : simulink/Logic and Bit Operations/Compare To Zero  relop=~=  OutDataTypeStr=boolean
  Constant : Constant
  Data Type Conversion : DataTypeConversion
  Data Type Conversion1 : DataTypeConversion  OutDataTypeStr=uint16
  Data Type Conversion2 : DataTypeConversion
  Display : Display
      settings: Format=hex (Stored Integer)
  Divide : Product  Inputs=**
  Shift Arithmetic : ArithShift  BitShiftNumber=8  BitShiftDirection=Right
  Switch : Switch  Criteria=u2 > Threshold
  LowByte : Outport  VectorParamsAs1DForOutWhenUnconnected=off
  HighByte : Outport  Port=2  VectorParamsAs1DForOutWhenUnconnected=off
  wires:
  Compare To Zero/1 -> Switch/2
  Factor/1 -> Switch/1, Compare To Zero/1
  Data Type Conversion2/1 -> HighByte/1
  Data Type Conversion/1 -> LowByte/1
  Constant/1 -> Switch/3
  Switch/1 -> Divide/2
  Bitwise Operator/1 -> Shift Arithmetic/1
  Offset/1 -> Add/2
  Shift Arithmetic/1 -> Data Type Conversion2/1
  Bitwise Operator1/1 -> Data Type Conversion/1
  Data Type Conversion1/1 -> Bitwise Operator/1, Display/1, Bitwise Operator1/1
  Divide/1 -> Add/1
  Data/1 -> Divide/1
  Add/1 -> Data Type Conversion1/1

== system EPT/Foreground_TimeBase_5ms/CAN/CAN3_exec/HyPer9_MCU/RPDO4/Convert_Data2Byte1 ==
  Data : Inport
  Factor : Inport  Port=2
  Offset : Inport  Port=3
  Add : Sum
  Bitwise Operator : simulink/Logic and Bit Operations/Bitwise Operator  logicop=AND  UseBitMask=on  BitMask=bin2dec('1111111100000000')  BitMaskRealWorld=Stored Integer
  Bitwise Operator1 : simulink/Logic and Bit Operations/Bitwise Operator  logicop=AND  UseBitMask=on  BitMask=bin2dec('0000000011111111')  BitMaskRealWorld=Stored Integer
  Compare To Zero : simulink/Logic and Bit Operations/Compare To Zero  relop=~=  OutDataTypeStr=boolean
  Constant : Constant
  Data Type Conversion : DataTypeConversion
  Data Type Conversion1 : DataTypeConversion  OutDataTypeStr=uint16
  Data Type Conversion2 : DataTypeConversion
  Display : Display
      settings: Format=hex (Stored Integer)
  Divide : Product  Inputs=**
  Shift Arithmetic : ArithShift  BitShiftNumber=8  BitShiftDirection=Right
  Switch : Switch  Criteria=u2 > Threshold
  LowByte : Outport  VectorParamsAs1DForOutWhenUnconnected=off
  HighByte : Outport  Port=2  VectorParamsAs1DForOutWhenUnconnected=off
  wires:
  Add/1 -> Data Type Conversion1/1
  Data/1 -> Divide/1
  Divide/1 -> Add/1
  Data Type Conversion1/1 -> Bitwise Operator1/1, Display/1, Bitwise Operator/1
  Bitwise Operator1/1 -> Data Type Conversion/1
  Shift Arithmetic/1 -> Data Type Conversion2/1
  Offset/1 -> Add/2
  Bitwise Operator/1 -> Shift Arithmetic/1
  Switch/1 -> Divide/2
  Constant/1 -> Switch/3
  Data Type Conversion/1 -> LowByte/1
  Data Type Conversion2/1 -> HighByte/1
  Factor/1 -> Compare To Zero/1, Switch/1
  Compare To Zero/1 -> Switch/2

== system EPT/Foreground_TimeBase_5ms/CAN/CAN3_exec/HyPer9_MCU/TPDO1/Convert_Byte2Data ==
  LowByte : Inport
  HighByte : Inport  Port=2
  Offset : Inport  Port=3
  Factor : Inport  Port=4
  Add2 : Sum
  Add5 : Sum
  Compare To Zero : simulink/Logic and Bit Operations/Compare To Zero  relop===  OutDataTypeStr=boolean
  Constant1 : Constant
  Constant10 : Constant  Value=256
  Data Type Conversion1 : DataTypeConversion  OutDataTypeStr=int16
  Data Type Conversion10 : DataTypeConversion  OutDataTypeStr=double
  Divide6 : Product  Inputs=**
  Divide9 : Product  Inputs=**
  Switch : Switch  Criteria=u2 > Threshold
  Data : Outport  VectorParamsAs1DForOutWhenUnconnected=off
  wires:
  Constant1/1 -> Switch/1
  Factor/1 -> Compare To Zero/1, Switch/3
  Compare To Zero/1 -> Switch/2
  Switch/1 -> Divide9/2
  Divide6/1 -> Add2/2
  Add5/1 -> Data Type Conversion10/1
  Constant10/1 -> Divide6/2
  Divide9/1 -> Add5/1
  Add2/1 -> Data Type Conversion1/1
  Data Type Conversion10/1 -> Data/1
  Offset/1 -> Add5/2
  HighByte/1 -> Divide6/1
  LowByte/1 -> Add2/1
  Data Type Conversion1/1 -> Divide9/1

== system EPT/Foreground_TimeBase_5ms/CAN/CAN3_exec/HyPer9_MCU/TPDO1/Convert_Byte2Data1 ==
  LowByte : Inport
  HighByte : Inport  Port=2
  Offset : Inport  Port=3
  Factor : Inport  Port=4
  Add2 : Sum
  Add5 : Sum
  Compare To Zero : simulink/Logic and Bit Operations/Compare To Zero  relop===  OutDataTypeStr=boolean
  Constant1 : Constant
  Constant10 : Constant  Value=256
  Data Type Conversion1 : DataTypeConversion  OutDataTypeStr=int16
  Data Type Conversion10 : DataTypeConversion  OutDataTypeStr=double
  Divide6 : Product  Inputs=**
  Divide9 : Product  Inputs=**
  Switch : Switch  Criteria=u2 > Threshold
  Data : Outport  VectorParamsAs1DForOutWhenUnconnected=off
  wires:
  Data Type Conversion1/1 -> Divide9/1
  LowByte/1 -> Add2/1
  HighByte/1 -> Divide6/1
  Offset/1 -> Add5/2
  Data Type Conversion10/1 -> Data/1
  Add2/1 -> Data Type Conversion1/1
  Divide9/1 -> Add5/1
  Constant10/1 -> Divide6/2
  Add5/1 -> Data Type Conversion10/1
  Divide6/1 -> Add2/2
  Switch/1 -> Divide9/2
  Compare To Zero/1 -> Switch/2
  Factor/1 -> Switch/3, Compare To Zero/1
  Constant1/1 -> Switch/1

== system EPT/Foreground_TimeBase_5ms/CAN/CAN3_exec/HyPer9_MCU/TPDO1/Convert_Byte2Data2 ==
  LowByte : Inport
  HighByte : Inport  Port=2
  Offset : Inport  Port=3
  Factor : Inport  Port=4
  Add2 : Sum
  Add5 : Sum
  Compare To Zero : simulink/Logic and Bit Operations/Compare To Zero  relop===  OutDataTypeStr=boolean
  Constant1 : Constant
  Constant10 : Constant  Value=256
  Data Type Conversion1 : DataTypeConversion  OutDataTypeStr=int16
  Data Type Conversion10 : DataTypeConversion  OutDataTypeStr=double
  Divide6 : Product  Inputs=**
  Divide9 : Product  Inputs=**
  Switch : Switch  Criteria=u2 > Threshold
  Data : Outport  VectorParamsAs1DForOutWhenUnconnected=off
  wires:
  Constant1/1 -> Switch/1
  Factor/1 -> Compare To Zero/1, Switch/3
  Compare To Zero/1 -> Switch/2
  Switch/1 -> Divide9/2
  Divide6/1 -> Add2/2
  Add5/1 -> Data Type Conversion10/1
  Constant10/1 -> Divide6/2
  Divide9/1 -> Add5/1
  Add2/1 -> Data Type Conversion1/1
  Data Type Conversion10/1 -> Data/1
  Offset/1 -> Add5/2
  HighByte/1 -> Divide6/1
  LowByte/1 -> Add2/1
  Data Type Conversion1/1 -> Divide9/1

== system EPT/Foreground_TimeBase_5ms/CAN/CAN3_exec/HyPer9_MCU/TPDO1/Mains State  ==
  Byte : Inport
  Compare To Constant : simulink/Logic and Bit Operations/Compare To Constant  relop===  const=1  OutDataTypeStr=boolean
  Compare To Constant1 : simulink/Logic and Bit Operations/Compare To Constant  relop===  const=2  OutDataTypeStr=boolean
  Compare To Constant2 : simulink/Logic and Bit Operations/Compare To Constant  relop===  const=3  OutDataTypeStr=boolean
  Compare To Constant3 : simulink/Logic and Bit Operations/Compare To Constant  relop===  const=4  OutDataTypeStr=boolean
  Compare To Constant4 : simulink/Logic and Bit Operations/Compare To Constant  relop===  const=5  OutDataTypeStr=boolean
  Compare To Constant5 : simulink/Logic and Bit Operations/Compare To Constant  relop===  const=6  OutDataTypeStr=boolean
  Compare To Constant6 : simulink/Logic and Bit Operations/Compare To Constant  relop===  const=7  OutDataTypeStr=boolean
  Startup : Outport
  Mains Checking : Outport  Port=2
  Mains OK : Outport  Port=3
  Pre-Charging : Outport  Port=4
  Pre-Charge Done : Outport  Port=5
  "Power Ready " : Outport  Port=6
  "Alarmed " : Outport  Port=7
  wires:
  Byte/1 -> Compare To Constant/1, Compare To Constant1/1, Compare To Constant2/1, Compare To Constant3/1, Compare To Constant4/1, Compare To Constant5/1, Compare To Constant6/1
  Compare To Constant1/1 -> Mains Checking/1
  Compare To Constant2/1 -> Mains OK/1
  Compare To Constant3/1 -> Pre-Charging/1
  Compare To Constant4/1 -> Pre-Charge Done/1
  Compare To Constant5/1 -> "Power Ready "/1
  Compare To Constant6/1 -> "Alarmed "/1
  Compare To Constant/1 -> Startup/1

== system EPT/Foreground_TimeBase_5ms/CAN/CAN3_exec/HyPer9_MCU/TPDO2/Convert_Byte2Data ==
  LowByte : Inport
  HighByte : Inport  Port=2
  Offset : Inport  Port=3
  Factor : Inport  Port=4
  Add2 : Sum
  Add5 : Sum
  Compare To Zero : simulink/Logic and Bit Operations/Compare To Zero  relop===  OutDataTypeStr=boolean
  Constant1 : Constant
  Constant10 : Constant  Value=256
  Data Type Conversion1 : DataTypeConversion  OutDataTypeStr=int16
  Data Type Conversion10 : DataTypeConversion  OutDataTypeStr=double
  Divide6 : Product  Inputs=**
  Divide9 : Product  Inputs=**
  Switch : Switch  Criteria=u2 > Threshold
  Data : Outport  VectorParamsAs1DForOutWhenUnconnected=off
  wires:
  Data Type Conversion1/1 -> Divide9/1
  LowByte/1 -> Add2/1
  HighByte/1 -> Divide6/1
  Offset/1 -> Add5/2
  Data Type Conversion10/1 -> Data/1
  Add2/1 -> Data Type Conversion1/1
  Divide9/1 -> Add5/1
  Constant10/1 -> Divide6/2
  Add5/1 -> Data Type Conversion10/1
  Divide6/1 -> Add2/2
  Switch/1 -> Divide9/2
  Compare To Zero/1 -> Switch/2
  Factor/1 -> Switch/3, Compare To Zero/1
  Constant1/1 -> Switch/1

== system EPT/Foreground_TimeBase_5ms/CAN/CAN3_exec/HyPer9_MCU/TPDO2/Convert_Byte2Data1 ==
  LowByte : Inport
  HighByte : Inport  Port=2
  Offset : Inport  Port=3
  Factor : Inport  Port=4
  Add2 : Sum
  Add5 : Sum
  Compare To Zero : simulink/Logic and Bit Operations/Compare To Zero  relop===  OutDataTypeStr=boolean
  Constant1 : Constant
  Constant10 : Constant  Value=256
  Data Type Conversion1 : DataTypeConversion  OutDataTypeStr=int16
  Data Type Conversion10 : DataTypeConversion  OutDataTypeStr=double
  Divide6 : Product  Inputs=**
  Divide9 : Product  Inputs=**
  Switch : Switch  Criteria=u2 > Threshold
  Data : Outport  VectorParamsAs1DForOutWhenUnconnected=off
  wires:
  Constant1/1 -> Switch/1
  Factor/1 -> Compare To Zero/1, Switch/3
  Compare To Zero/1 -> Switch/2
  Switch/1 -> Divide9/2
  Divide6/1 -> Add2/2
  Add5/1 -> Data Type Conversion10/1
  Constant10/1 -> Divide6/2
  Divide9/1 -> Add5/1
  Add2/1 -> Data Type Conversion1/1
  Data Type Conversion10/1 -> Data/1
  Offset/1 -> Add5/2
  HighByte/1 -> Divide6/1
  LowByte/1 -> Add2/1
  Data Type Conversion1/1 -> Divide9/1

== system EPT/Foreground_TimeBase_5ms/CAN/CAN3_exec/HyPer9_MCU/TPDO2/Convert_Byte2Data2 ==
  LowByte : Inport
  HighByte : Inport  Port=2
  Offset : Inport  Port=3
  Factor : Inport  Port=4
  Add2 : Sum
  Add5 : Sum
  Compare To Zero : simulink/Logic and Bit Operations/Compare To Zero  relop===  OutDataTypeStr=boolean
  Constant1 : Constant
  Constant10 : Constant  Value=256
  Data Type Conversion1 : DataTypeConversion  OutDataTypeStr=int16
  Data Type Conversion10 : DataTypeConversion  OutDataTypeStr=double
  Divide6 : Product  Inputs=**
  Divide9 : Product  Inputs=**
  Switch : Switch  Criteria=u2 > Threshold
  Data : Outport  VectorParamsAs1DForOutWhenUnconnected=off
  wires:
  Data Type Conversion1/1 -> Divide9/1
  LowByte/1 -> Add2/1
  HighByte/1 -> Divide6/1
  Offset/1 -> Add5/2
  Data Type Conversion10/1 -> Data/1
  Add2/1 -> Data Type Conversion1/1
  Divide9/1 -> Add5/1
  Constant10/1 -> Divide6/2
  Add5/1 -> Data Type Conversion10/1
  Divide6/1 -> Add2/2
  Switch/1 -> Divide9/2
  Compare To Zero/1 -> Switch/2
  Factor/1 -> Switch/3, Compare To Zero/1
  Constant1/1 -> Switch/1
